simulink model "SensorSimulinkVehicle"  (R2024a)
settings: Solver=FixedStepAuto  StartTime=0  StopTime=1000  FixedStep=simStepSize  RelTol=1e-3
PreLoadFcn:
  | % To support Reader and Writer blocks, some bus objects must be loaded
  | loadRoadRunnerBusObject();
undefined symbols (not defined in the file or in its folder): gainArg, simStepSize
libraries: drivingscenarioandsensors x1, roadrunnerscenario x1
settings Model: Creator=The MathWorks, Inc.  LastModifiedBy=fukuchi
settings SolverCC: MaxZcPerStep=1
settings DataIOCC: SaveOutput=off  DSMLogging=off  SaveTime=off  ReturnWorkspaceOutputs=off
settings ModelReferenceCC: EnableRefExpFcnMdlSchedulingChecks=on
settings RTWCC: GPUComputeCapability=3.5  DLArmComputeVersion=19.05

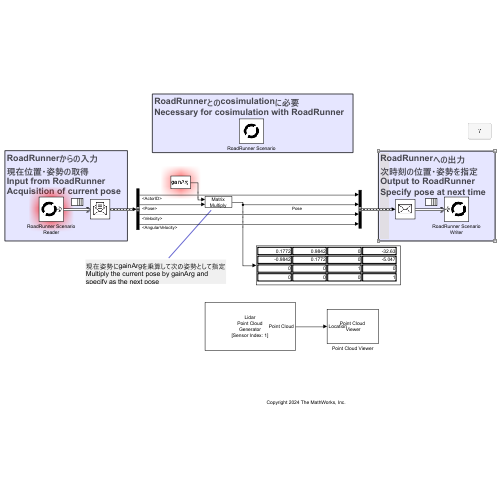
[thumbnail: Simulink's stored preview of the top-level diagram]
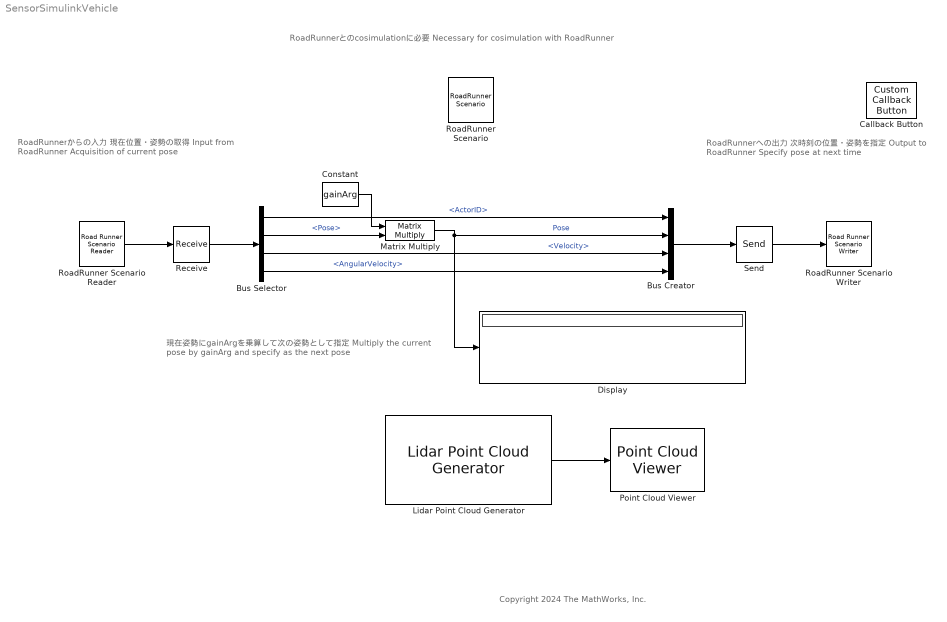
== system SensorSimulinkVehicle ==
  note: 現在姿勢にgainArgを乗算して次の姿勢として指定
      | Multiply the current pose by gainArg and specify as the next pose
  note: RoadRunnerとのcosimulationに必要
      | Necessary for cosimulation with RoadRunner
  note: Copyright 2024 The MathWorks, Inc.
  note: RoadRunnerからの入力
      | 現在位置・姿勢の取得
      | Input from RoadRunner
      | Acquisition of current pose
  note: RoadRunnerへの出力
      | 次時刻の位置・姿勢を指定
      | Output to RoadRunner
      | Specify pose at next time
  Bus Creator : BusCreator  Inputs=4  OutDataTypeStr=Bus: BusActorRuntime  NonVirtualBus=on
  Bus Selector : BusSelector  OutputSignals=ActorID,Pose,Velocity,AngularVelocity
  Callback Button : CustomCallbackButton  Configuration="{\"components\":[{\"name\":\"BackgroundImageComponent\",\"settings\":{\"image\":{\"size\":[0,0],\"src\":\"default\",\"srcOrientation\":\"Right\"},\"position\":[0,0,1,1]}},{\"name\":\"ButtonStateComponent\",\"settings\":{\"buttonType\":\"momentary\",\"clickFcn\":\"helpview('driving','SimulateRoadRunnerwithSimulink')\",\"onValue\":1,\"position\":[0,0,1,1],\"pressDelay\":\"500\",\"pressFcn\":\"\",\"repeatInterval\":\"0\",\"states\":[{\"horizontalAlignment\":\"center\",\"image\":{\"position\":[0,0,1,1],\"src\":\"default\",\"srcOrientation\":\"Right\"},\"label\":{\"color\":[0.01176470588,0.01176470588,0.01176470588,1],\"icon\":{\"size\":[0,0],\"src\":\"default\",\"srcOrientation\":\"Right\"},\"iconPlacement\":\"left\",\"text\":{\"content\":\"?\"}},\"labelOffset\":[0,0],\"verticalAlignment\":\"middle\"},{\"horizontalAlignment\":\"center\",\"image\":{\"position\":[0,0,1,1],\"src\":\"default\",\"srcOrientation\":\"Right\"},\"label\":{\"color\":[0.01176470588,0.01176470588,0.01176470588,1],\"icon\":{\"size\":[0,0],\"src\":\"default\",\"srcOrientation\":\"Right\"},\"iconPlacement\":\"left\",\"text\":{\"content\":\"?\"}},\"labelOffset\":[0,0],\"verticalAlignment\":\"middle\"},{\"horizontalAlignment\":\"center\",\"image\":{\"position\":[0,0,1,1],\"src\":\"default\",\"srcOrientation\":\"Right\"},\"label\":{\"color\":[0.01176470588,0.01176470588,0.01176470588,1],\"icon\":{\"size\":[0,0],\"src\":\"default\",\"srcOrientation\":\"Right\"},\"iconPlacement\":\"left\",\"text\":{\"content\":\"?\"}},\"labelOffset\":[0,0],\"verticalAlignment\":\"middle\"},{\"horizontalAlignment\":\"center\",\"image\":{\"position\":[0,0,1,1],\"src\":\"default\",\"srcOrientation\":\"Right\"},\"label\":{\"color\":[0.01176470588,0.01176470588,0.01176470588,1],\"icon\":{\"size\":[0,0],\"src\":\"default\",\"srcOrientation\":\"Right\"},\"iconPlacement\":\"left\",\"text\":{\"content\":\"?\"}},\"labelOffset\":[0,0],\"verticalAlignment\":\"middle\"}]}},{\"name\":\"ForegroundImageComponent\",\"settings\":{\"image\":{\"size\":[0,0],\"src\":\"default\",\"srcOrientation\":\"Right\"},\"isForeground\":1,\"position\":[0,0,1,1]}}],\"settings\":{\"BindingType\":\"standalone\",\"backgroundColor\":[244,244,244,1],\"backgroundOffset\":0.2,\"backgroundOpacity\":1,\"fixedAspectRatio\":\"off\",\"foregroundColor\":[0.01176470588,0.01176470588,0.01176470588,1],\"migratedFromLegacy\":true,\"useBackgroundColor\":true,\"variant\":\"callback\",\"version\":\"R2023a\"},\"type\":\"Button\"}"  CustomBackgroundColor="{\"color\":[0.9568627451,0.9568627451,0.9568627451],\"show\":true}"
  Constant : Constant  Value=gainArg  VectorParams1D=off
  Display : Display
  Lidar Point Cloud Generator : drivingscenarioandsensors/Lidar Point Cloud Generator  SensorIndex=1  UpdateInterval=0.1  SensorLocation=[1.5 0]  Height=1.6  Yaw=0  Pitch=0  Roll=0  DetectionCoordinates=Ego Cartesian  HasEgoVehicle=on  EgoVehicleActorID=2  HasRoadsInputPort=on  ActorProfilesSource=From Scenario Reader block  ActorProfilesVariableName=actor_profiles  MaxRange=120  RangeAccuracy=0.002  AzimuthResolution=0.16  ElevationResolution=1.25  AzimuthLimits=[ -180, 180 ]  ElevationLimits=[ -20, 20 ]  HasNoise=on
  Matrix Multiply : Product  Multiplication=Matrix(*)
  Point Cloud Viewer : PointCloudViewer  FigPos=[1028 668 874 359]
  Receive : Receive  InputPortMessageModes=m  UseInternalQueue=off  QueueOverwriting=on  QueueLength=1  QueueType=LIFO
  RoadRunner Scenario : roadrunnerscenario/RoadRunner Scenario  UserDefinedActions={}  UserDefinedEvents={}
  RoadRunner Scenario Reader : RoadRunnerScenarioReader  OutputPortMessageModes=m  TopicType=Actor Pose  VehicleType=Vehicle Specifications  SampleTime=simStepSize
  RoadRunner Scenario Writer : RoadRunnerScenarioWriter  InputPortMessageModes=m  TopicType=Actor Pose  VehicleType=Vehicle Pose
  Send : Send  OutputPortMessageModes=m
  wires:
  RoadRunner Scenario Reader/1 -> Receive/1
  Receive/1 -> Bus Selector/1
  Bus Creator/1 -> Send/1
  Bus Selector/1 -> Bus Creator/1  "<ActorID>"
  Bus Selector/4 -> Bus Creator/4  "<AngularVelocity>"
  Bus Selector/2 -> Matrix Multiply/2  "<Pose>"
  Constant/1 -> Matrix Multiply/1
  Matrix Multiply/1 -> Bus Creator/2, Display/1  "Pose"
  Send/1 -> RoadRunner Scenario Writer/1
  Bus Selector/3 -> Bus Creator/3  "<Velocity>"
  Lidar Point Cloud Generator/1 -> Point Cloud Viewer/1
